simulink model "PC_Quadcopter_Simulation_Hexacopter_health_wind"  (R2022b)
settings: Solver=ode4  StartTime=0.0  StopTime=100  FixedStep=0.01  MaxStep=0.06  RelTol=1e-3
PreLoadFcn:
  | DoB_parameter
model workspace (MAT data in the model file):
  Sig = Simulink.Signal
  Sig.DataType = 'auto'
  Sig.Dimensions = -1
  Sig.DimensionsMode = 'auto'
  Sig.Complexity = 'auto'
  Sig.SampleTime = -1
  Sig.SamplingMode = 'auto'
values from neighbouring files (symbols this model uses):
  A = [ ... (first row only)    [DoB_parameter.m]
  B = [0 1 0]'    [DoB_parameter.m]
  C = [1 0 0]    [DoB_parameter.m]
  den_Inv_X = conv(num_X,den_Qfilter)    [DoB_parameter.m]
  den_Inv_Y = conv(num_Y, den_Qfilter)    [DoB_parameter.m]
  den_Inv_Z = conv(num_Z, den_Qfilter_Z)    [DoB_parameter.m]
  den_Qfilter = [1 a1/tau a0/tau^2]    [DoB_parameter.m]
  den_Qfilter_Z = [1 a1/tau a0/tau^2]    [DoB_parameter.m]
  I_xx = J(1,1)    [DoB_parameter.m]
  I_yy = J(2,2)    [DoB_parameter.m]
  I_zz = J(3,3)    [DoB_parameter.m]
  IC = block.DialogPrm(2).Data    [quadcopterDynamicsSFunction.m]
  L = [l1 l2 l3]'    [DoB_parameter.m]
  num_Inv_X = conv(den_X,num_Qfilter)    [DoB_parameter.m]
  num_Inv_Y = conv(den_Y, num_Qfilter)    [DoB_parameter.m]
  num_Inv_Z = conv(den_Z, num_Qfilter_Z)    [DoB_parameter.m]
  num_Qfilter = a0/tau^2    (= 100)    [DoB_parameter.m]
  num_Qfilter_Z = a0/tau^2    (= 11.1111111111)    [DoB_parameter.m]
undefined symbols (not defined in the file or in its folder): F, Light, magnitude, MIL, quadModel
libraries: simulink x37, sharedTrackingLibrary x1, aerolibwind2 x1
(part 1 of 3)
Description:
  | This is a configurable quadcopter simulation.
  | This Simulink model demonstates position control.
  | 
  | Additional quadcopter modeling and simulation materials available at:
  | github.com/dch33/Quad-Sim
  | 
  | Copyright (C) 2014 D. Hartman, K. Landis, S. Moreno, J. Kim, M. Mehrer
  | 
  | License:
  |     This program is free software: you can redistribute it and/or modify
  |     it under the terms of the GNU LESSER GENERAL PUBLIC LICENSE as published by
  |     the Free Software Foundation, either version 3 of the License, or
  |     (at your option) any later version.
  | 
  |     This program is distributed in the hope that it will be useful,
  |     but WITHOUT ANY WARRANTY; without even the implied warranty of
  |     MERCHANTABILITY or FITNESS FOR A PARTICULAR PURPOSE.  See the
  |     GNU General Public License for more details.
  | 
  |     You should have received a copy of the GNU LESSER GENERAL PUBLIC LICENSE
  |     along with this program.  If not, see <http://www.gnu.org/licenses/>.
settings Model: ModifiedComment=skim -- Tue May 01 16:43:25 2018 -- Version 1.6  Creator=David Hartman  LastModifiedBy=박범준
settings Model: ModifiedHistory=|
  | skim -- Tue May 01 16:43:25 2018 -- Version 1.6
  | 
  | 
  | davidhartman -- Fri Jun 06 22:59:54 2014 -- Version 1.5
settings SolverCC: AlgebraicLoopSolver=TrustRegion
settings DataIOCC: SaveFormat=Array  SignalLogging=off  ReturnWorkspaceOutputs=off
settings OptimizationCC: DefaultParameterBehavior=Inlined  LifeSpan=inf
settings DebuggingCC: SolverPrmCheckMsg=warning  UnconnectedInputMsg=warning  UnconnectedOutputMsg=warning  UnconnectedLineMsg=warning  UniqueDataStoreMsg=warning  StateNameClashWarn=warning  StrictBusMsg=ErrorOnBusTreatedAsVector  SFUnexpectedBacktrackingDiag=warning  SFNoUnconditionalDefaultTransitionDiag=warning  SFExecutionAtInitializationDiag=none  SFMachineParentedDataDiag=warning  ArithmeticOperatorsInVariantConditions=warning
settings HardwareCC: ProdBitPerPointer=32  ProdBitPerSizeT=32  ProdBitPerPtrDiffT=32  ProdLargestAtomicFloat=None  ProdIntDivRoundTo=Undefined  ProdEndianess=Unspecified  ProdWordSize=32  ProdHWDeviceType=32-bit Generic
settings ModelReferenceCC: EnableRefExpFcnMdlSchedulingChecks=on  PropagateSignalLabelsOutOfModel=off
settings SFSimCC: SimUseLocalCustomCode=off  CustomCodeUndefinedFunction=UseInterfaceOnly
settings RTWCC: RTWUseLocalCustomCode=off  DLArmComputeVersion=19.05
settings CodeAppCC: StateflowObjectComments=on
settings GRTTargetCC: TargetLangStandard=C89/C90 (ANSI)
settings ConfigComp: CovMetricSettings=dw  CovSaveCumulativeToWorkspaceVar=on  CovSaveSingleToWorkspaceVar=on  CovExternalEMLEnable=off

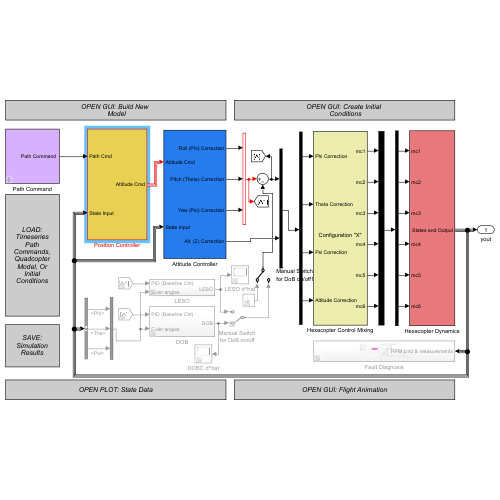
[thumbnail: Simulink's stored preview of the top-level diagram]
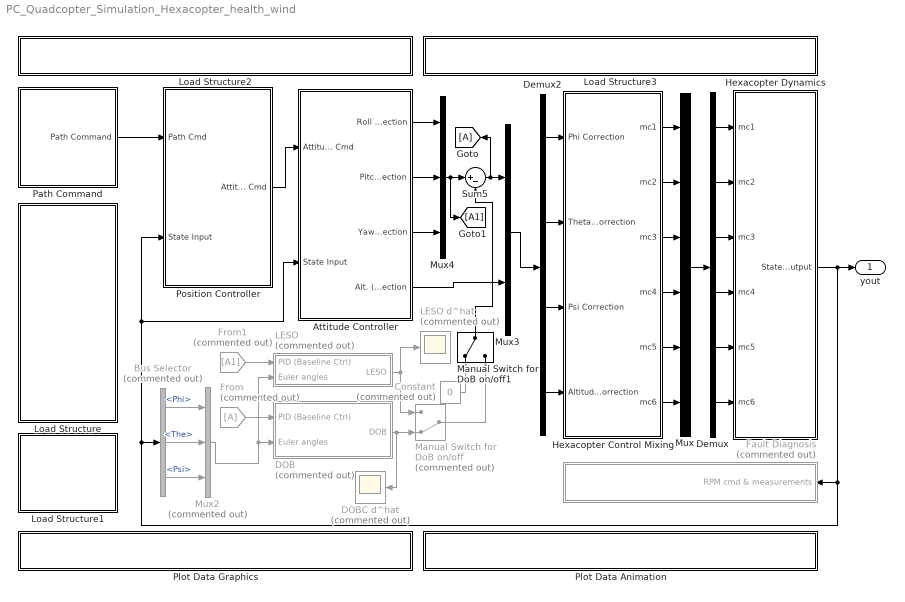
== system PC_Quadcopter_Simulation_Hexacopter_health_wind ==
  Attitude Controller : Subsystem
  Bus Selector : BusSelector  Commented=on  OutputSignals=Phi,The,Psi
  Constant : Constant  Commented=on  Value=0
  DOB : Subsystem  Commented=on
  DOBC d^hat : Scope  Commented=on
  Demux : Demux  Outputs=6
  Demux2 : Demux
  Fault Diagnosis : Subsystem  Commented=on
  From : From  Commented=on
  From1 : From  Commented=on  GotoTag=A1
  Goto : Goto
  Hexacopter Control Mixing : Subsystem
      mask Display:
      | modelLoaded = evalin('base','exist(''quadModel'',''var'')');
      | if (modelLoaded==1)
      |     if (evalin('base','quadModel.plusConfig'))
      |     fprintf([' \n' ' \n'  'Configuration "+"']);
      |     else if (~evalin('base','quadModel.plusConfig'))
      |         fprintf([' \n' ' \n' 'Configuration "X"']);
      |         end
      |     end
      | else
      |     fprintf([' \n' ' \n'  'Model Not Loaded']);
      | end
  Hexacopter Dynamics : Subsystem
  LESO : Subsystem  Commented=on
  LESO d^hat : Scope  Commented=on
  Load Structure : Subsystem
      settings: OpenFcn=|
      | uiopen('load')
      | if ((exist('IC')==1) && (exist('quadModel')==1) && (exist('path')==1))
      | set_param(bdroot, 'SimulationCommand', 'update')
      | end
      mask Display: fprintf('LOAD:\nTimeseries\nPath\nCommands,\nQuadcopter\nModel, Or\nInitial\nConditions');
  Load Structure1 : Subsystem
      settings: OpenFcn=|
      | if (exist('IC')==1 && exist('quadModel')==1 && exist('yout') && exist('tout'))
      | saveSimResults()
      | else
      | msgbox('No Data To Save!')
      | end
      mask Display: fprintf('SAVE:\nSimulation\nResults');
  Load Structure2 : Subsystem
      settings: OpenFcn=|
      | if exist('GUI_Modeling') == 2,
      | run('GUI_Modeling')
      | 
      | else
      | 
      | msgbox('The desired GUI must be first added to MATLABs path.')
      | 
      | end
      mask Display: fprintf('OPEN GUI: Build New \n Model');
  Load Structure3 : Subsystem
      settings: OpenFcn=|
      | if exist('GUI_IC') == 2,
      | run('GUI_IC')
      | 
      | else
      | 
      | msgbox('The desired GUI must be first added to MATLABs path.')
      | 
      | end
      mask Display: fprintf('OPEN GUI: Create Initial \n Conditions');
  Manual Switch for DoB on/off : ManualSwitch  Commented=on  CurrentSetting=0
  Manual Switch for DoB on/off1 : ManualSwitch
  Mux : Mux  Inputs=6
  Mux2 : Mux  Commented=on  Inputs=3
  Mux3 : Mux  Inputs=2
  Mux4 : Mux  Inputs=3
  Path Command : Subsystem  mask{Interpolate=off, OutputAfterFinalValue=Holding final value}
      mask prompts: Interpolate "Interpolate X, Y, Z, and Psi command data?"; OutputAfterFinalValue "Form output after final data value by:"
      mask help:
      | Selecting the Interpolate data checkbox causes position commands to be
      | linearly interpolated. For additional options related to the Timeseries
      | "path" commands, look under the block and click on the Timeseries From
      | Workspace blocks.
      mask TypeOptions Interpolate: X Timeseries From Wkspace/Interpolate | Y Timeseries From Wkspace/Interpolate | Z Timeseries From Wkspace/Interpolate | Psi Timeseries From Wkspace/Interpolate
      mask TypeOptions OutputAfterFinalValue: X Timeseries From Wkspace/OutputAfterFinalValue | Y Timeseries From Wkspace/OutputAfterFinalValue | Z Timeseries From Wkspace/OutputAfterFinalValue | Psi Timeseries From Wkspace/OutputAfterFinalValue
  Plot Data Animation : Subsystem
      settings: OpenFcn=|
      | if exist('QuadAnim4') == 2,
      |     if exist('yout')
      | 	run('QuadAnim4');
      |     else
      |     msgbox('Simulation must be run before data can be plotted.');
      |     end
      | else                                                                          msgbox('The desired GUI must be first added to MATLABs path.')
      | end
      mask Display: fprintf('OPEN GUI: Flight Animation')
  Plot Data Graphics : Subsystem
      settings: OpenFcn=|
      | if exist('yout')
      | yout = evalin('base', 'yout');
      | tout = evalin('base', 'tout');
      | quadPlots(yout, tout)
      | else
      | msgbox('Simulation must be run before data can be plotted.')
      | end
      mask Display: fprintf('OPEN PLOT: State Data')
  Position Controller : Subsystem
  Sum5 : Sum  Inputs=|+-
  yout : Outport
  wires:
  Hexacopter Dynamics/1(States and Output) -> yout/1, Position Controller/2(State Input), Attitude Controller/2(State Input), Bus Selector/1, Fault Diagnosis/1(RPM cmd & measurements)
  Position Controller/1(Attitude Cmd) -> Attitude Controller/1(Attitude Cmd)
  Mux/1 -> Demux/1
  Hexacopter Control Mixing/2(mc2) -> Mux/2
  Hexacopter Control Mixing/3(mc3) -> Mux/3
  Hexacopter Control Mixing/1(mc1) -> Mux/1
  Hexacopter Control Mixing/4(mc4) -> Mux/4
  Demux/3 -> Hexacopter Dynamics/3(mc3)
  Demux/4 -> Hexacopter Dynamics/4(mc4)
  Demux/1 -> Hexacopter Dynamics/1(mc1)
  Demux/2 -> Hexacopter Dynamics/2(mc2)
  Attitude Controller/3(Yaw (Psi) Correction) -> Mux4/3
  Attitude Controller/1(Roll (Phi) Correction) -> Mux4/1
  Attitude Controller/2(Pitch (Theta) Correction) -> Mux4/2
  Demux2/3 -> Hexacopter Control Mixing/3(Psi Correction)
  Demux2/4 -> Hexacopter Control Mixing/4(Altitude Correction)
  Demux2/2 -> Hexacopter Control Mixing/2(Theta Correction)
  Demux2/1 -> Hexacopter Control Mixing/1(Phi Correction)
  DOB/1(DOB) -> DOBC d^hat/1, Manual Switch for DoB on/off/2
  Bus Selector/2 -> Mux2/2  "<The>"
  Bus Selector/3 -> Mux2/3  "<Psi>"
  Bus Selector/1 -> Mux2/1  "<Phi>"
  Mux2/1 -> LESO/2(Euler angles), DOB/2(Euler angles)
  From/1 -> DOB/1(PID (Baseline Ctrl))
  Mux4/1 -> [A1], Sum5/1
  Sum5/1 -> Goto/1, Mux3/1
  Attitude Controller/4(Alt. (Z) Correction) -> Mux3/2
  Mux3/1 -> Demux2/1
  Manual Switch for DoB on/off/1 -> Manual Switch for DoB on/off1/2
  Manual Switch for DoB on/off1/1 -> Sum5/2
  LESO/1(LESO) -> LESO d^hat/1, Manual Switch for DoB on/off/1
  From1/1 -> LESO/1(PID (Baseline Ctrl))
  Hexacopter Control Mixing/5(mc5) -> Mux/5
  Hexacopter Control Mixing/6(mc6) -> Mux/6
  Demux/5 -> Hexacopter Dynamics/5(mc5)
  Demux/6 -> Hexacopter Dynamics/6(mc6)
  Constant/1 -> Manual Switch for DoB on/off1/1
  Path Command/1("Path Command ") -> Position Controller/1(Path Cmd)

== system PC_Quadcopter_Simulation_Hexacopter_health_wind/Attitude Controller ==
  Attitude Cmd : Inport
  State Input : Inport  Port=2
  Altitude (Z) Control : Subsystem  mask{Kpz=9, Kiz=6.6, Kdz=9.9, LimitOutput=on, USat=1, LSat=-1, GOffset=(sqrt((quadModel.mass*quadModel.g)/(6*quadModel.ct))-quadModel.b)/quadModel.cr}
      mask prompts: Kpz "Kp"; Kiz "Ki"; Kdz "Kd"; LimitOutput "Integral Saturation?"; USat "Upper saturation limit:"; LSat "Lower saturation limit:"; GOffset "Gravity Feedforward"
      mask help:
      | Adjust PID controller gains through this mask interface, or "look under mask" for more detailed adjustments.
      |
      | Note: Gravity Offset will not appear on block face as a value until simulation is run if it is the result of a formula involving the quadcopter model parameters.
      mask TypeOptions Kpz: Kpz/Gain
      mask TypeOptions Kiz: Kiz/Gain
      mask TypeOptions Kdz: Kdz/Gain
      mask TypeOptions LimitOutput:
      | Integrator
      | Limited/LimitOutput
      mask TypeOptions USat:
      | Integrator
      | Limited/UpperSaturationLimit
      mask TypeOptions LSat:
      | Integrator
      | Limited/LowerSaturationLimit
      mask TypeOptions GOffset: Gravity Offset (Level Flight)/Value
      mask Display:
      | fprintf(['Gravity Offset = ' num2str(GOffset) '\n' ...
      |     'Kp = ' num2str(Kpz) '\n' ...
      |     'Ki = ' num2str(Kiz) '\n' ...
      |     'Kd = ' num2str(Kdz) '\n' ...
      |     'Integral Saturation: ' LimitOutput]);
      | if strcmp(LimitOutput,'on')
      |     fprintf([' \n' ' \n' ' \n' ' \n' ' \n' '\n' ...
      |         'Limits: ' num2str(USat) ' to ' num2str(LSat)]);
      | end
  Bus Selector : BusSelector  OutputSignals=Phi,P,The,Q,Psi,R,Z
  Pitch (Theta) Control : Subsystem  mask{Kpt=2, Kit=1.1, Kdt=1.2, LimitOutput=on, USat=1, LSat=-1}
      mask prompts: Kpt "Kp"; Kit "Ki"; Kdt "Kd"; LimitOutput "Integral Saturation?"; USat "Upper saturation limit:"; LSat "Lower saturation limit:"
      mask help: Adjust PID controller gains through this mask interface, or "look under mask" for more detailed adjustments.
      mask TypeOptions Kpt: Kpt/Gain
      mask TypeOptions Kit: Kit/Gain
      mask TypeOptions Kdt: Kdt/Gain
      mask TypeOptions LimitOutput:
      | Integrator
      | Limited/LimitOutput
      mask TypeOptions USat:
      | Integrator
      | Limited/UpperSaturationLimit
      mask TypeOptions LSat:
      | Integrator
      | Limited/LowerSaturationLimit
      mask Display:
      | fprintf(['Kp = ' num2str(Kpt) '\n' ...
      |     'Ki = ' num2str(Kit) '\n' ...
      |     'Kd = ' num2str(Kdt) '\n' ...
      |     'Integral Saturation: ' LimitOutput]);
      | if strcmp(LimitOutput,'on')
      |     fprintf([' \n' ' \n' ' \n' ' \n' '\n' ...
      |         'Limits: ' num2str(USat) ' to ' num2str(LSat)]);
      | end
  "Roll (Phi) Control " : Subsystem  mask{Kpp=2, Kip=1.1, Kdp=1.2, LimitOutput=on, USat=1, LSat=-1}
      mask prompts: Kpp "Kp"; Kip "Ki"; Kdp "Kd"; LimitOutput "Integral Saturation:"; USat "Upper saturation limit:"; LSat "Lower saturation limit:"
      mask help:
      | Adjust PID controller gains through this mask interface, or "look under mask"
      | for more detailed adjustments.
      mask TypeOptions Kpp: Kpp/Gain
      mask TypeOptions Kip: Kip/Gain
      mask TypeOptions Kdp: Kdp/Gain
      mask TypeOptions LimitOutput:
      | Integrator
      | Limited/LimitOutput
      mask TypeOptions USat:
      | Integrator
      | Limited/UpperSaturationLimit
      mask TypeOptions LSat:
      | Integrator
      | Limited/LowerSaturationLimit
      mask Display:
      | fprintf(['Kp = ' num2str(Kpp) '\n' ...
      |     'Ki = ' num2str(Kip) '\n' ...
      |     'Kd = ' num2str(Kdp) '\n'...
      |     'Integral Saturation: ' LimitOutput]);
      | if strcmp(LimitOutput,'on')
      |     fprintf([' \n' ' \n' ' \n' ' \n' '\n' ...
      |         'Limits: ' num2str(USat) ' to ' num2str(LSat)]);
      | end
  Yaw (Psi) Control : Subsystem  mask{Kps=0.3, Kis=0.15, Kds=0.5, LimitOutput=on, USat=1, LSat=-1}
      mask prompts: Kps "Kp"; Kis "Ki"; Kds "Kd"; LimitOutput "Integral Saturation?"; USat "Upper saturation limit:"; LSat "Lower saturation limit:"
      mask help: Adjust PID controller gains through this mask interface, or "look under mask" for more detailed adjustments.
      mask TypeOptions Kps: Kps/Gain
      mask TypeOptions Kis: Kit/Gain
      mask TypeOptions Kds: Kds/Gain
      mask TypeOptions LimitOutput:
      | Integrator
      | Limited/LimitOutput
      mask TypeOptions USat:
      | Integrator
      | Limited/UpperSaturationLimit
      mask TypeOptions LSat:
      | Integrator
      | Limited/LowerSaturationLimit
      mask Display:
      | fprintf(['Kp = ' num2str(Kps) '\n' ...
      |     'Ki = ' num2str(Kis) '\n' ...
      |     'Kd = ' num2str(Kds) '\n' ...
      |     'Integral Saturation: ' LimitOutput]);
      | if strcmp(LimitOutput,'on')
      |     fprintf([' \n' ' \n' ' \n' ' \n' '\n' ...
      |         'Limits: ' num2str(USat) ' to ' num2str(LSat)]);
      | end
  Roll (Phi) Correction : Outport
  Pitch (Theta) Correction : Outport  Port=2
  Yaw (Psi) Correction : Outport  Port=3
  Alt. (Z) Correction : Outport  Port=4
  wires:
  "Roll (Phi) Control "/1(Phi Correction) -> Roll (Phi) Correction/1
  Bus Selector/1 -> "Roll (Phi) Control "/2(Phi State)  "<Phi>"
  State Input/1 -> Bus Selector/1
  Pitch (Theta) Control/1(Theta Correction) -> Pitch (Theta) Correction/1
  Yaw (Psi) Control/1(Psi Correction) -> Yaw (Psi) Correction/1
  Bus Selector/5 -> Yaw (Psi) Control/2(Psi State)  "<Psi>"
  Altitude (Z) Control/1(Alt. (Z) Correction) -> Alt. (Z) Correction/1
  Bus Selector/7 -> Altitude (Z) Control/2(Z State)  "<Z>"
  Attitude Cmd/1 -> Altitude (Z) Control/1(Desired Z), Yaw (Psi) Control/1(Attitude Command), Pitch (Theta) Control/1(Attitude Command), "Roll (Phi) Control "/1("Attitude Command ")
  Bus Selector/3 -> Pitch (Theta) Control/2(Theta State)  "<The>"
  Bus Selector/2 -> "Roll (Phi) Control "/3(P)  "<P>"
  Bus Selector/4 -> Pitch (Theta) Control/3(P State)  "<Q>"
  Bus Selector/6 -> Yaw (Psi) Control/3(R State)  "<R>"

== system PC_Quadcopter_Simulation_Hexacopter_health_wind/DOB ==
  PID (Baseline Ctrl) : Inport
  Euler angles : Inport  Port=2
  Demux : Demux  Outputs=3
  Demux1 : Demux  Outputs=3
  Mux : Mux  Inputs=3
  Subsystem : Subsystem
  Subsystem1 : Subsystem
  Subsystem2 : Subsystem
  DOB : Outport
  wires:
  PID (Baseline Ctrl)/1 -> Demux/1
  Euler angles/1 -> Demux1/1
  Demux/1 -> Subsystem/1(PID_X)
  Demux1/1 -> Subsystem/2(Angle_X)
  Demux/2 -> Subsystem1/1(PID_Y)
  Demux1/2 -> Subsystem1/2(Anlgel_Y)
  Demux/3 -> Subsystem2/1(PID_Z)
  Demux1/3 -> Subsystem2/2(Angle_Z)
  Subsystem/1(DOB_X) -> Mux/1
  Subsystem1/1(DOB_Y) -> Mux/2
  Subsystem2/1(DOB_Z) -> Mux/3
  Mux/1 -> DOB/1

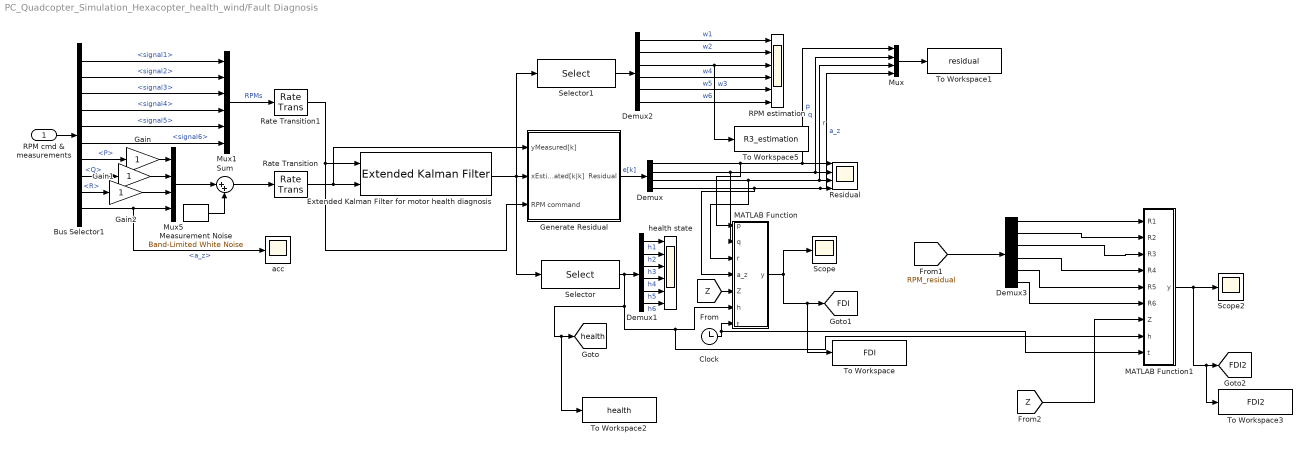
== system PC_Quadcopter_Simulation_Hexacopter_health_wind/Fault Diagnosis ==
  RPM cmd & measurements : Inport
  Bus Selector1 : BusSelector  OutputSignals=mc and RPM.signal1,mc and RPM.signal2,mc and RPM.signal3,mc and RPM.signal4,mc and RPM.signal5,mc and RPM.signal6,P,Q,R,a_z
  Clock : Clock
  Demux : Demux
  Demux1 : Demux  Outputs=6
  Demux2 : Demux  Outputs=6
  Demux3 : Demux  Outputs=6
  Extended Kalman Filter for motor health diagnosis : sharedTrackingLibrary/Extended Kalman Filter  StateTransitionFcn=myStateTransitionFcn  HasStateTransitionJacobianFcn=on  StateTransitionJacobianFcn=myStateJacobian  HasAdditiveProcessNoise=Additive  ProcessNoise=1e-2*diag(ones(15,1))  HasTimeVaryingProcessNoise=off  HasStateTransitionFcnExtraArgument=1  InitialState=[0;0;0;3360*ones(6,1);ones(6,1)]  InitialStateCovariance=1e-4*eye(15)  MeasurementFcn1=myMeasurementFcn  HasMeasurementJacobianFcn1=on  MeasurementJacobianFcn1=myMeasurementJacobian  HasMeasurementEnablePort1=off  HasAdditiveMeasurementNoise1=Additive  MeasurementNoise1=1e-4*diag(ones(4,1))  HasTimeVaryingMeasurementNoise1=off  HasMeasurementFcnExtraArgument1=0  HasMeasurementWrapping1=off  MeasurementFcn2=myMeasurementFcn  HasMeasurementJacobianFcn2=off  HasMeasurementEnablePort2=off  HasAdditiveMeasurementNoise2=Additive  MeasurementNoise2=1  HasTimeVaryingMeasurementNoise2=off  HasMeasurementFcnExtraArgument2=0  HasMeasurementWrapping2=off  MeasurementFcn3=myMeasurementFcn  HasMeasurementJacobianFcn3=off  HasMeasurementEnablePort3=off  HasAdditiveMeasurementNoise3=Additive  MeasurementNoise3=1  HasTimeVaryingMeasurementNoise3=off  HasMeasurementFcnExtraArgument3=0  HasMeasurementWrapping3=off  MeasurementFcn4=myMeasurementFcn  HasMeasurementJacobianFcn4=off  HasMeasurementEnablePort4=off  HasAdditiveMeasurementNoise4=Additive  MeasurementNoise4=1  HasTimeVaryingMeasurementNoise4=off  HasMeasurementFcnExtraArgument4=0  HasMeasurementWrapping4=off  MeasurementFcn5=myMeasurementFcn  HasMeasurementJacobianFcn5=off  HasMeasurementEnablePort5=off  HasAdditiveMeasurementNoise5=Additive  MeasurementNoise5=1  HasTimeVaryingMeasurementNoise5=off  HasMeasurementFcnExtraArgument5=0  HasMeasurementWrapping5=off  EnableMultirate=off  StateTransitionFcnSampleTime=1  MeasurementFcn1SampleTime=1  MeasurementFcn2SampleTime=1  MeasurementFcn3SampleTime=1  MeasurementFcn4SampleTime=1  MeasurementFcn5SampleTime=1  UseCurrentEstimator=on  OutputStateCovariance=off  DataType=double  SampleTime=0.05  NumberOfMeasurements=1
  Gain : Gain
  Gain1 : Gain
  Gain2 : Gain
  Generate Residual : Subsystem
  MATLAB Function : MATLAB Function  TreatAsAtomicUnit=on
  MATLAB Function1 : MATLAB Function  TreatAsAtomicUnit=on
  Measurement Noise : simulink/Sources/Band-Limited White Noise  Cov=[(1e-6)^2*ones(1,3) (1e-3)^2]  Ts=0.05  seed=[23342]
  Mux : Mux
  Mux1 : Mux  Inputs=6
  Mux5 : Mux
  RPM estimation : Scope  NumInputPorts=6
  Rate Transition : RateTransition  OutPortSampleTime=0.05
  Rate Transition1 : RateTransition  OutPortSampleTime=0.05
  Residual : Scope  NumInputPorts=4
  Scope : Scope
  Scope2 : Scope
  Selector : Selector  InputPortWidth=15  IndexOptions=Index vector (dialog)  Indices=[10:15]  OutputSizes=1
  Selector1 : Selector  InputPortWidth=15  IndexOptions=Index vector (dialog)  Indices=[4:9]  OutputSizes=1
  Sum : Sum  Inputs=|++
  To Workspace : ToWorkspace  VariableName=FDI  SampleTime=-1
  To Workspace1 : ToWorkspace  VariableName=residual  SampleTime=-1
  To Workspace2 : ToWorkspace  VariableName=health  SampleTime=-1
  To Workspace3 : ToWorkspace  VariableName=FDI2  SampleTime=-1
  To Workspace5 : ToWorkspace  VariableName=R3_estimation  SampleTime=-1
  acc : Scope
  health state : Scope  NumInputPorts=6
  tag scope: FDI2=global, FDI=global, health=global
  wires:
  Bus Selector1/1 -> Mux1/1  "<signal1>"
  Mux1/1 -> Rate Transition1/1  "RPMs"
  Rate Transition/1 -> Extended Kalman Filter for motor health diagnosis/2, Generate Residual/1(yMeasured[k])
  Bus Selector1/2 -> Mux1/2  "<signal2>"
  Bus Selector1/5 -> Mux1/5  "<signal5>"
  Bus Selector1/4 -> Mux1/4  "<signal4>"
  Bus Selector1/8 -> Gain1/1  "<Q>"
  Bus Selector1/3 -> Mux1/3  "<signal3>"
  Bus Selector1/9 -> Gain2/1  "<R>"
  Bus Selector1/10 -> acc/1, Mux5/4  "<a_z>"
  Bus Selector1/7 -> Gain/1  "<P>"
  Extended Kalman Filter for motor health diagnosis/1 -> Selector1/1, Selector/1, Generate Residual/2(xEstimated[k|k])
  Bus Selector1/6 -> Mux1/6  "<signal6>"
  Mux5/1 -> Sum/1
  Sum/1 -> Rate Transition/1
  RPM cmd & measurements/1 -> Bus Selector1/1
  Rate Transition1/1 -> Generate Residual/3(RPM command), Extended Kalman Filter for motor health diagnosis/1
  Generate Residual/1(Residual) -> Demux/1  "e[k]"
  Demux/1 -> MATLAB Function/1(p), Mux/1, Residual/1  "p"
  Demux/2 -> MATLAB Function/2(q), Mux/2, Residual/2  "q"
  Demux/3 -> MATLAB Function/3(r), Mux/3, Residual/3  "r"
  Demux/4 -> MATLAB Function/4(a_z), Mux/4, Residual/4  "a_z"
  Selector/1 -> MATLAB Function1/8(h), MATLAB Function/6(h), To Workspace2/1, [health], Demux1/1
  Demux1/1 -> health state/1  "h1"
  Demux1/2 -> health state/2  "h2"
  Demux1/3 -> health state/3  "h3"
  Demux1/4 -> health state/4  "h4"
  Demux1/5 -> health state/5  "h5"
  Demux1/6 -> health state/6  "h6"
  Demux2/3 -> To Workspace5/1, RPM estimation/3  "w3"
  Demux2/4 -> RPM estimation/4  "w4"
  Demux2/2 -> RPM estimation/2  "w2"
  Demux2/5 -> RPM estimation/5  "w5"
  Demux2/6 -> RPM estimation/6  "w6"
  Selector1/1 -> Demux2/1
  Demux2/1 -> RPM estimation/1  "w1"
  Measurement Noise/1 -> Sum/2
  Gain/1 -> Mux5/1
  Gain1/1 -> Mux5/2
  Gain2/1 -> Mux5/3
  MATLAB Function/1(y) -> Scope/1, To Workspace/1, [FDI]
  [Z] -> MATLAB Function/5(Z)
  Clock/1 -> MATLAB Function1/9(t), MATLAB Function/7(t)
  Mux/1 -> To Workspace1/1
  [Z] -> MATLAB Function1/7(Z)
  MATLAB Function1/1(y) -> To Workspace3/1, [FDI2], Scope2/1
  [RPM_residual] -> Demux3/1
  Demux3/1 -> MATLAB Function1/1(R1)
  Demux3/2 -> MATLAB Function1/2(R2)
  Demux3/3 -> MATLAB Function1/3(R3)
  Demux3/4 -> MATLAB Function1/4(R4)
  Demux3/5 -> MATLAB Function1/5(R5)
  Demux3/6 -> MATLAB Function1/6(R6)

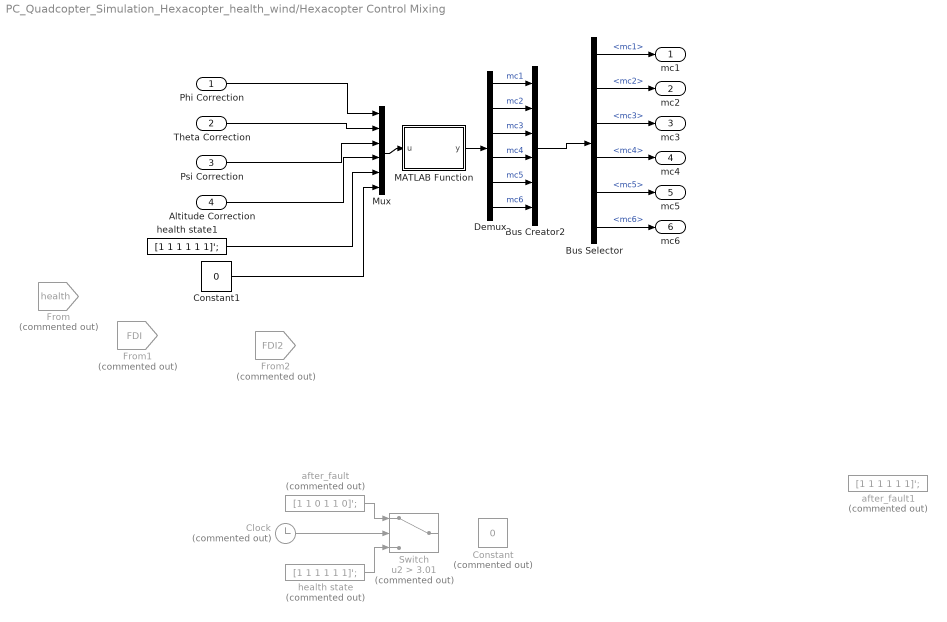
== system PC_Quadcopter_Simulation_Hexacopter_health_wind/Hexacopter Control Mixing ==
  Phi Correction : Inport
  Theta Correction : Inport  Port=2
  Psi Correction : Inport  Port=3
  Altitude Correction : Inport  Port=4
  Bus Creator2 : BusCreator  Inputs=6
  Bus Selector : BusSelector  OutputSignals=mc1,mc2,mc3,mc4,mc5,mc6
  Clock : Clock  Commented=on
  Constant : Constant  Commented=on  Value=0
  Constant1 : Constant  Value=0
  Demux : Demux  Outputs=6
  From : From  Commented=on  GotoTag=health  TagVisibility=global
  From1 : From  Commented=on  GotoTag=FDI  TagVisibility=global
  From2 : From  Commented=on  GotoTag=FDI2  TagVisibility=global
  MATLAB Function : MATLAB Function  TreatAsAtomicUnit=on
  Mux : Mux  Inputs=6
  Switch : Switch  Commented=on  Criteria=u2 > Threshold  Threshold=3.01  SaturateOnIntegerOverflow=off  InputSameDT=off
  after_fault : Constant  Commented=on  Value=[1 1 0 1 1 0]';
  after_fault1 : Constant  Commented=on  Value=[1 1 1 1 1 1]';
  health state : Constant  Commented=on  Value=[1 1 1 1 1 1]';
  health state1 : Constant  Value=[1 1 1 1 1 1]';
  mc1 : Outport
  mc2 : Outport  Port=2
  mc3 : Outport  Port=3
  mc4 : Outport  Port=4
  mc5 : Outport  Port=5
  mc6 : Outport  Port=6
  wires:
  Phi Correction/1 -> Mux/1
  Theta Correction/1 -> Mux/2
  Psi Correction/1 -> Mux/3
  Altitude Correction/1 -> Mux/4
  Bus Selector/1 -> mc1/1  "<mc1>"
  Bus Selector/2 -> mc2/1  "<mc2>"
  Bus Selector/3 -> mc3/1  "<mc3>"
  Bus Selector/4 -> mc4/1  "<mc4>"
  Bus Selector/5 -> mc5/1  "<mc5>"
  Bus Selector/6 -> mc6/1  "<mc6>"
  Mux/1 -> MATLAB Function/1(u)
  MATLAB Function/1(y) -> Demux/1
  Demux/6 -> Bus Creator2/6  "mc6"
  Demux/3 -> Bus Creator2/3  "mc3"
  Demux/4 -> Bus Creator2/4  "mc4"
  Demux/1 -> Bus Creator2/1  "mc1"
  Demux/5 -> Bus Creator2/5  "mc5"
  Demux/2 -> Bus Creator2/2  "mc2"
  Bus Creator2/1 -> Bus Selector/1
  Constant1/1 -> Mux/6
  health state1/1 -> Mux/5
  health state/1 -> Switch/3
  after_fault/1 -> Switch/1
  Clock/1 -> Switch/2

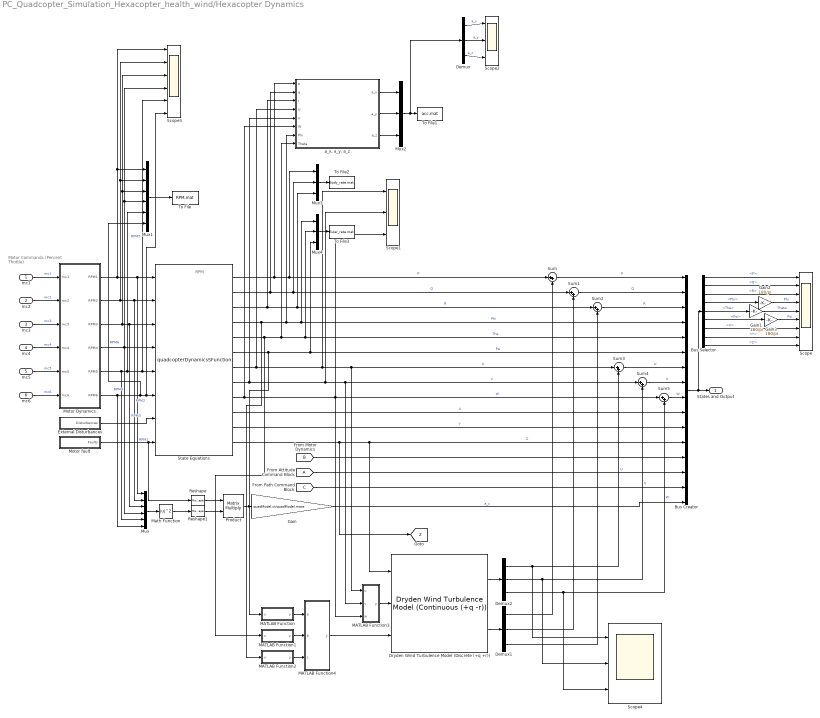
== system PC_Quadcopter_Simulation_Hexacopter_health_wind/Hexacopter Dynamics ==
  note: RPM
  note: Motor Commands
      | (Percent Thottle)
  mc1 : Inport
  mc2 : Inport  Port=2
  mc3 : Inport  Port=3
  mc4 : Inport  Port=4
  mc5 : Inport  Port=5
  mc6 : Inport  Port=6
  Bus Creator : BusCreator  Inputs=P,Q,R,Phi,The,Psi,U,V,W,X,Y,Z,mc and RPM,Attitude_Cmd,XY_Cmd,a_z
  Bus Selector : BusSelector  OutputSignals=P,Q,R,Phi,The,Psi,X,Y,Z
  Demux : Demux  Outputs=3
  Demux1 : Demux  Outputs=3
  Demux2 : Demux  Outputs=3
  Dryden Wind Turbulence Model (Discrete (+q +r)) : aerolibwind2/Dryden Wind Turbulence Model  (Continuous (+q -r))  units=Metric (MKS)  spec=MIL-F-8785C  model=Discrete Dryden (+q +r)  W20=3  Wdeg=0  TurbProb=10^-2 - Light  L_high=533.4  Wingspan=1  ts=0.1  Seed=[23341 23342 23343 23344]  T_on=on
      settings: LibrarySourceBlock=|
      | aerolibwind2/Dryden Wind Turbulence Model
      | (Discrete (+q +r))
  External Disturbances : Subsystem
  From Attitude Command Block : From  TagVisibility=global
  Gain : Gain  Gain=quadModel.ct/quadModel.mass
  Gain1 : Gain  Gain=180/pi
  Gain2 : Gain  Gain=180/pi
  Gain3 : Gain  Gain=180/pi
  MATLAB Function : MATLAB Function  TreatAsAtomicUnit=on
  MATLAB Function1 : MATLAB Function  TreatAsAtomicUnit=on
  MATLAB Function2 : MATLAB Function  TreatAsAtomicUnit=on
  MATLAB Function3 : MATLAB Function  TreatAsAtomicUnit=on
  MATLAB Function4 : MATLAB Function  TreatAsAtomicUnit=on
  Math Function : Math  Operator=magnitude^2
  Motor Dynamics : Subsystem
  Motor fault : Subsystem
  Mux : Mux  Inputs=6
  Mux1 : Mux  Inputs=6
  Mux2 : Mux  Inputs=3
  Mux3 : Mux  Inputs=3
  Mux4 : Mux  Inputs=3
  Product : Product  Multiplication=Matrix(*)
  Reshape : Reshape  OutputDimensionality=Row vector (2-D)
  Reshape1 : Reshape  OutputDimensionality=Column vector (2-D)
  Scope : Scope  NumInputPorts=9
  Scope1 : Scope  NumInputPorts=3
  Scope2 : Scope  NumInputPorts=3
  Scope3 : Scope  NumInputPorts=6
  Scope4 : Scope  NumInputPorts=3
  State Equations : M-S-Function  FunctionName=quadcopterDynamicsSFunction  Parameters=quadModel, IC
      mask Display:
      | port_label('input', 1, 'RPM1')
      | port_label('input', 2, 'RPM2')
      | port_label('input', 3, 'RPM3')
      | port_label('input', 4, 'RPM4')
      | port_label('input', 5, 'RPM5')
      | port_label('input', 6, 'RPM6')
      | port_label('input', 7, 'Disturbances')
      | port_label('input', 8, 'Faults')
      | port_label('output', 1, 'P')
      | port_label('output', 2, 'Q')
      | port_label('output', 3, 'R')
      | port_label('output', 4, 'Phi')
      | port_label('output', 5, 'The')
      | port_label('output', 6, 'Psi')
      | port_label('output', 7, 'U')
      | port_label('output', 8, 'V')
      | port_label('output', 9, 'W')
      | port_label('output', 10, 'X')
      | port_label('output', 11, 'Y')
      | port_label('output', 12, 'Z')
  Sum{,1..5} (6 alike) : Sum  Inputs=|++
  To File : ToFile  Filename=RPM.mat  MatrixName=RPM  SaveFormat=Timeseries
  To File1 : ToFile  Filename=acc.mat  MatrixName=acc  SaveFormat=Timeseries
  To File2 : ToFile  Filename=Body_rate.mat  MatrixName=Body_rate  SaveFormat=Timeseries
  To File3 : ToFile  Filename=Euler_rate.mat  MatrixName=Euler_rate  SaveFormat=Timeseries
  "a_x, a_y, a_z" : Subsystem
  States and Output : Outport
  tag scope: Z=global
  wires:
  State Equations/1 -> "a_x, a_y, a_z"/1(p), Sum/1, Mux3/1  "P"
  State Equations/2 -> "a_x, a_y, a_z"/2(q), Sum1/1, Mux3/2  "Q"
  State Equations/3 -> "a_x, a_y, a_z"/3(r), Sum2/1, Mux3/3  "R"
  State Equations/4 -> MATLAB Function2/1(u), "a_x, a_y, a_z"/7(Phi), Mux4/1, Bus Creator/4  "Phi"
  State Equations/5 -> MATLAB Function1/1(u), "a_x, a_y, a_z"/8(Theta), Mux4/2, Bus Creator/5  "The"
  State Equations/6 -> MATLAB Function/1(u), Bus Creator/6, Mux4/3  "Psi"
  State Equations/7 -> "a_x, a_y, a_z"/4(U), MATLAB Function3/1(u), Sum3/1, Scope1/1  "U"
  State Equations/8 -> "a_x, a_y, a_z"/5(V), MATLAB Function3/2(v), Sum4/1, Scope1/2  "V"
  State Equations/9 -> "a_x, a_y, a_z"/6(W), MATLAB Function3/3(w), Scope1/3, Sum5/1  "W"
  State Equations/10 -> Bus Creator/10  "X"
  State Equations/11 -> Bus Creator/11  "Y"
  State Equations/12 -> Dryden Wind Turbulence Model (Discrete (+q +r))/1, Bus Creator/12, [Z]  "Z"
  Bus Creator/1 -> Bus Selector/1, States and Output/1
  Motor Dynamics/1(RPM1) -> Scope3/1, Mux1/1, Mux/1, State Equations/1  "RPM1"
  Motor Dynamics/2(RPM2) -> Mux1/2, Scope3/2, Mux/2, State Equations/2  "RPM2"
  Motor Dynamics/3(RPM3) -> Mux1/3, Scope3/3, State Equations/3, Mux/3  "RPM3"
  Motor Dynamics/4(RPM4) -> Mux1/4, Scope3/4, Mux/4, State Equations/4  "RPM4"
  mc1/1 -> Motor Dynamics/1(mc1)  "mc1"
  mc4/1 -> Motor Dynamics/4(mc4)  "mc4"
  mc3/1 -> Motor Dynamics/3(mc3)  "mc3"
  mc2/1 -> Motor Dynamics/2(mc2)  "mc2"
  External Disturbances/1("Disturbances ") -> State Equations/7
  From Attitude Command Block/1 -> Bus Creator/14
  [B] -> Bus Creator/13
  [C] -> Bus Creator/15
  mc5/1 -> Motor Dynamics/5(mc5)  "mc5"
  mc6/1 -> Motor Dynamics/6(mc6)  "mc6"
  Motor Dynamics/5(RPM5) -> Mux/5, Mux1/5, Scope3/5, State Equations/5  "RPM5"
  Motor Dynamics/6(RPM6) -> Mux/6, Mux1/6, Scope3/6, State Equations/6  "RPM6"
  Motor fault/1(Faults) -> Reshape/1, State Equations/8
  Bus Selector/1 -> Scope/1  "<P>"
  Bus Selector/2 -> Scope/2  "<Q>"
  Bus Selector/3 -> Scope/3  "<R>"
  Bus Selector/4 -> Gain2/1  "<Phi>"
  Bus Selector/5 -> Gain1/1  "<The>"
  Bus Selector/6 -> Gain3/1  "<Psi>"
  Bus Selector/7 -> Scope/7  "<X>"
  Bus Selector/8 -> Scope/8  "<Y>"
  Bus Selector/9 -> Scope/9  "<Z>"
  Mux/1 -> Math Function/1
  Math Function/1 -> Reshape1/1
  Product/1 -> Gain/1
  Reshape/1 -> Product/1
  Reshape1/1 -> Product/2
  Gain/1 -> Bus Creator/16  "a_z"
  Gain1/1 -> Scope/5  "Theta"
  Gain2/1 -> Scope/4  "Phi"
  Gain3/1 -> Scope/6  "Psi"
  Mux1/1 -> To File/1
  "a_x, a_y, a_z"/2(a_y) -> Mux2/2
  "a_x, a_y, a_z"/1(a_x) -> Mux2/1
  "a_x, a_y, a_z"/3(a_z) -> Mux2/3
  Mux2/1 -> Demux/1, To File1/1
  Demux/1 -> Scope2/1  "a_x"
  Demux/2 -> Scope2/2  "a_y"
  Demux/3 -> Scope2/3  "a_z"
  Mux3/1 -> To File2/1
  Mux4/1 -> To File3/1
  Dryden Wind Turbulence Model (Discrete (+q +r))/2 -> Demux1/1
  Dryden Wind Turbulence Model (Discrete (+q +r))/1 -> Demux2/1
  MATLAB Function/1(y) -> MATLAB Function4/1(a)
  MATLAB Function1/1(y) -> MATLAB Function4/2(b)
  MATLAB Function2/1(y) -> MATLAB Function4/3(c)
  MATLAB Function4/1(y) -> Dryden Wind Turbulence Model (Discrete (+q +r))/3
  Demux1/1 -> Sum/2
  Demux1/2 -> Sum1/2
  Demux1/3 -> Sum2/2
  Sum1/1 -> Bus Creator/2  "Q"
  Sum/1 -> Bus Creator/1  "P"
  Sum2/1 -> Bus Creator/3  "R"
  Demux2/1 -> Scope4/1, Sum3/2  "U"
  Demux2/2 -> Scope4/2, Sum4/2  "V"
  Sum3/1 -> Bus Creator/7  "U"
  Sum4/1 -> Bus Creator/8  "V"
  Sum5/1 -> Bus Creator/9  "W"
  MATLAB Function3/1(y) -> Dryden Wind Turbulence Model (Discrete (+q +r))/2
  Demux2/3 -> Scope4/3, Sum5/2  "W"

== system PC_Quadcopter_Simulation_Hexacopter_health_wind/LESO ==
  PID (Baseline Ctrl) : Inport
  Euler angles : Inport  Port=2
  Demux : Demux  Outputs=3
  Demux1 : Demux  Outputs=3
  Gain : Gain  Gain=I_xx
  Gain1 : Gain  Gain=I_yy
  Gain2 : Gain  Gain=I_zz
  Gain4 : Gain  Gain=1/I_xx
  Gain5 : Gain  Gain=1/I_yy
  Gain6 : Gain  Gain=1/I_zz
  Linear Extended-State Observer : Subsystem
  Linear Extended-State Observer1 : Subsystem
  Linear Extended-State Observer2 : Subsystem
  Mux : Mux  Inputs=3
  LESO : Outport
  wires:
  Mux/1 -> LESO/1
  Euler angles/1 -> Demux1/1
  PID (Baseline Ctrl)/1 -> Demux/1
  Demux1/1 -> Linear Extended-State Observer/1(y)
  Demux/1 -> Gain4/1
  Linear Extended-State Observer/2(x3_hat (F)) -> Gain/1
  Demux1/2 -> Linear Extended-State Observer1/1(y)
  Demux/2 -> Gain5/1
  Linear Extended-State Observer1/2(x3_hat (F)) -> Gain1/1
  Demux1/3 -> Linear Extended-State Observer2/1(y)
  Demux/3 -> Gain6/1
  Linear Extended-State Observer2/2(x3_hat (F)) -> Gain2/1
  Gain/1 -> Mux/1
  Gain1/1 -> Mux/2
  Gain2/1 -> Mux/3
  Gain4/1 -> Linear Extended-State Observer/2(u)
  Gain5/1 -> Linear Extended-State Observer1/2(u)
  Gain6/1 -> Linear Extended-State Observer2/2(u)

== system PC_Quadcopter_Simulation_Hexacopter_health_wind/Load Structure ==

== system PC_Quadcopter_Simulation_Hexacopter_health_wind/Load Structure1 ==

== system PC_Quadcopter_Simulation_Hexacopter_health_wind/Load Structure2 ==

== system PC_Quadcopter_Simulation_Hexacopter_health_wind/Load Structure3 ==

== system PC_Quadcopter_Simulation_Hexacopter_health_wind/Path Command ==
  Bus Creator : BusCreator  Inputs=4
  Bus Selector : BusSelector  OutputSignals=X_cmd,Y_cmd  OutputAsBus=on
  Psi Timeseries From Wkspace : FromWorkspace  VariableName=path.psi  Interpolate=off  OutputAfterFinalValue=Holding final value
  X Timeseries From Wkspace : FromWorkspace  VariableName=path.x  Interpolate=off  OutputAfterFinalValue=Holding final value
  Y Timeseries From Wkspace : FromWorkspace  VariableName=path.y  Interpolate=off  OutputAfterFinalValue=Holding final value
  Z Timeseries From Wkspace : FromWorkspace  VariableName=path.z  Interpolate=off  OutputAfterFinalValue=Holding final value
  "Path Command " : Outport
  tag scope: C=global
  wires:
  X Timeseries From Wkspace/1 -> Bus Creator/1  "X_cmd"
  Y Timeseries From Wkspace/1 -> Bus Creator/2  "Y_cmd"
  Z Timeseries From Wkspace/1 -> Bus Creator/3  "Alt_Cmd"
  Psi Timeseries From Wkspace/1 -> Bus Creator/4  "Psi_cmd"
  Bus Creator/1 -> Bus Selector/1, "Path Command "/1  "Path_Cmd"
  Bus Selector/1 -> [C]  "XY_Cmd"

== system PC_Quadcopter_Simulation_Hexacopter_health_wind/Plot Data Animation ==

== system PC_Quadcopter_Simulation_Hexacopter_health_wind/Plot Data Graphics ==
